simulink model "planner_contral"  (R2023b)
settings: Solver=FixedStepAuto  StartTime=0  StopTime=inf  FixedStep=0.001  RelTol=1e-3
undefined symbols (not defined in the file): aubr, c_factor, cf, cr, iniObsHeading1, iniObsHeading2, iniObsPos1, iniObsPos2, KD_PID_distance, KD_PID_speed, KI_PID_distance, KI_PID_speed, KP_PID_distance, KP_PID_speed, la, lb, LQR_K1, LQR_K2, LQR_K3, LQR_K4, m, rack_displacement, refInfo_obs1, refInfo_obs2, right_wheel_ground, rightWaypoints, tablebr, vubr, vx_break_point
libraries: Solver_SF x1
(part 4 of 8)

== matlab function planner_contral/decision_planning/EMplanner/obs/Cartesian2Frenet_dynamic/location transformer ==
  data: x_set input; s_set output; y_set input; frenet_path_x input; frenet_path_y input; proj_x_set input; proj_y_set input; proj_heading_set input; proj_match_point_index_set input; index2s input; l_set output
function [s_set,l_set] = fcn(x_set,y_set,frenet_path_x,frenet_path_y,...
    proj_x_set,proj_y_set,proj_heading_set,proj_match_point_index_set,index2s)
    %该函数将计算世界坐标系下的x_set，y_set上的点在frenet_path下的坐标s l
    %输入 x_set,y_set 待坐标转换的点
    %     frenet_path_x,frenet_path_y   frenet坐标轴
    %     proj_x,y,heading,kappa,proj_match_point_index 待坐标转换的点的投影点的信息
    %     index2s   frenet_path的index与s的转换表

    % 由于不知道有多少个点需要做坐标转换，所以需要做缓冲
    n = 128;%最多处理128个点
    %输出初始化
    s_set = ones(n,1)*nan;
    l_set = ones(n,1)*nan;
    for i = 1:length(x_set)
        if isnan(x_set(i))
            break;
        end
        %计算s，写个子函数
        s_set(i) = CalcSFromIndex2S(index2s,frenet_path_x,frenet_path_y,proj_x_set(i),proj_y_set(i),...
            proj_match_point_index_set(i));
        n_r = [-sin(proj_heading_set(i));cos(proj_heading_set(i))];
        r_h = [x_set(i);y_set(i)];
        r_r = [proj_x_set(i);proj_y_set(i)];
        l_set(i) = (r_h - r_r)'*n_r;
    end
end

function s = CalcSFromIndex2S(index2s,path_x,path_y,proj_x,proj_y,proj_match_point_index)
  %该函数将计算当指定index2s的映射关系后，计算点proj_x,proj_y的弧长
  vector_1 = [proj_x;proj_y] - [path_x(proj_match_point_index);path_y(proj_match_point_index)];
  %这里要考虑的更全面一些，因为要考虑到proj_match_point_index有可能在path的起点或终点
  if (proj_match_point_index < length(path_x))
      vector_2 = [path_x(proj_match_point_index + 1);path_y(proj_match_point_index + 1)] - ...
          [path_x(proj_match_point_index);path_y(proj_match_point_index)];
  else
      vector_2 = [path_x(proj_match_point_index);path_y(proj_match_point_index)] - ...
          [path_x(proj_match_point_index - 1);path_y(proj_match_point_index - 1)];
  end
  
  if vector_1'*vector_2 > 0
      s = index2s(proj_match_point_index) + sqrt(vector_1'*vector_1);
  else
      s = index2s(proj_match_point_index) - sqrt(vector_1'*vector_1);
  end
  
  
end

== matlab function planner_contral/decision_planning/EMplanner/obs/Cartesian2Frenet_dynamic/velocity transformer ==
  data: l_set input; s_dot_set output; vx_set input; vy_set input; proj_heading_set input; proj_kappa_set input; l_dot_set output; dl_set output
function [s_dot_set,l_dot_set,dl_set] = fcn(l_set,vx_set,vy_set,proj_heading_set,proj_kappa_set)
%该函数将计算frenet坐标系下的s_dot, l_dot, dl/ds
n = 128;
% 输出初始化
s_dot_set = ones(n,1)*nan;
l_dot_set = ones(n,1)*nan;
dl_set = ones(n,1)*nan;

for i = 1 : length(l_set)
    if isnan(l_set(i))
        break;
    end
    v_h = [vx_set(i);vy_set(i)];
    n_r = [-sin(proj_heading_set(i));cos(proj_heading_set(i))];
    t_r = [cos(proj_heading_set(i));sin(proj_heading_set(i))];
    l_dot_set(i) = v_h'*n_r;
    s_dot_set(i) = v_h'*t_r/(1 - proj_kappa_set(i)*l_set(i));
    %%%向量法做cartesian与frenet的转换要更简单，但是也有缺点，向量法必须依赖速度加速度
    %l' = l_dot/s_dot 但是如果s_dot = 0 此方法就失效了
    if abs(s_dot_set(i)) < 1e-6
        dl_set(i) = 0;
    else
        dl_set(i) = l_dot_set(i)/s_dot_set(i);
    end
end

== matlab function planner_contral/decision_planning/EMplanner/obs/Cartesian2Frenet_dynamic/acc transformer ==
  data: ax_set input; s_dot2_set output; ay_set input; proj_heading_set input; proj_kappa_set input; l_set input; s_dot_set input; dl_set input; l_dot2_set output; ddl_set output
function [s_dot2_set,l_dot2_set,ddl_set] = fcn(ax_set,ay_set,proj_heading_set,proj_kappa_set,l_set,s_dot_set,dl_set)
%由于不知道有多少个点需要做坐标转换，设一个最大值做缓冲
n = 128;
% 输出初始化
s_dot2_set = ones(n,1)*nan;
l_dot2_set = ones(n,1)*nan;
ddl_set = ones(n,1)*nan;

for i = 1:length(l_set)
    if isnan(l_set(i))
       break;
    end
    a_h = [ax_set(i);ay_set(i)];
    n_r = [-sin(proj_heading_set(i));cos(proj_heading_set(i))];
    t_r = [cos(proj_heading_set(i));sin(proj_heading_set(i))];
    %近似认为dkr/ds 为0 简化计算
    l_dot2_set(i) = a_h'*n_r - proj_kappa_set(i) * (1 - proj_kappa_set(i) * l_set(i)) * s_dot_set(i)^2;
    s_dot2_set(i) = (1/(1 - proj_kappa_set(i) * l_set(i)))* (a_h' * t_r + 2 * proj_kappa_set(i) * dl_set(i) * s_dot_set(i)^2);
    % 要考虑加速度为0的情况
    if (s_dot2_set(i) < 1e-6)
        ddl_set(i) = 0;
    else
        ddl_set(i) = (l_dot2_set(i) - dl_set(i)*s_dot2_set(i))/(s_dot_set(i)^2);
    end
end

== matlab function planner_contral/decision_planning/EMplanner/path planning task/generate convex space ==
  data: dp_path_s input; l_min output; dp_path_l input; static_obs_s_set input; static_obs_l_set input; dynamic_obs_s input; dynamic_obs_l input; dynamic_obs_heading input; l_max output; obs_length input; obs_width input
function [l_min,l_max] = fcn(dp_path_s,dp_path_l,static_obs_s_set,static_obs_l_set,dynamic_obs_s,dynamic_obs_l,dynamic_obs_heading,obs_length,obs_width)
    % 该函数将输出每个离散的dp_path_s所对应的l的边界lmin lmax (本质上是质点的凸空间)
    % 输入 动态规划曲线 dp_path_s,dp_path_l
    %      障碍物中心的s l 坐标 static_obs_s,static_obs_l
    %      障碍物的长宽 static_obs_length,static_obs_width 
    % 输出 l_min lmax l 的上下界

    % 输出初始化
    l_min = ones(60,1) * -8;
    l_max = ones(60,1) * 8;
    % 对每个静态障碍物做遍历
    for i = 1:length(static_obs_s_set)
        if isnan(static_obs_s_set(i))
            break;
        end
        % 计算障碍物的头部和尾部的s
        obs_s_min = static_obs_s_set(i) - obs_length/2;
        obs_s_max = static_obs_s_set(i) + obs_length/2;
        % 找到dp_path_s 中，与s_head s_end最近的s的编号
        start_index = FindNearIndex(dp_path_s,obs_s_min);
        end_index = FindNearIndex(dp_path_s,obs_s_max);
        path_l = (dp_path_l(start_index) + dp_path_l(end_index))/2;
        if start_index == 1 && end_index == 1
            continue;
        end
        if path_l > static_obs_l_set(i)
            % 意味着决策为向左绕过障碍物
            for j = start_index:end_index
                % l_min(j) 为所有决策为向左绕过障碍物的l边界的最大值
                l_min(j) = max(l_min(j) , static_obs_l_set(i) + obs_width/2+0.6);
            end
        else
            % 意味着决策为向右绕过障碍物
            for j = start_index:end_index
                % l_max(j) 为所有决策为向右绕过障碍物的l边界的最小值
                l_max(j) = min(l_max(j) ,static_obs_l_set(i) - obs_width/2-0.6);
            end
        end       
    end
%计算动态障碍物的上界与下界
for i=1:length(dynamic_obs_s)
    if isnan(dynamic_obs_s(i))
        break;
    end
    %计算障碍物的头和尾，通过障碍物的坐标点及其航向角计算
%         obs_s_min = dynamic_obs_s(i) - obs_length/2;
%         obs_s_max = dynamic_obs_s(i) + obs_length/2;
        [l_max_,l_min_,s_max_,s_min_]=getboxpoint(dynamic_obs_s(i),dynamic_obs_l(i),dynamic_obs_heading(i),obs_length,obs_width);
        obs_s_min =s_min_;
        obs_s_max=s_max_;
        obs_l_min=l_min_;
        obs_l_max=l_max_;
        start_index = FindNearIndex(dp_path_s,obs_s_min);
        end_index = FindNearIndex(dp_path_s,obs_s_max);
        path_l = (dp_path_l(start_index) + dp_path_l(end_index))/2;
        if start_index == 1 && end_index == 1
            continue;
        end
         if path_l > dynamic_obs_l(i)
            % 意味着决策为向左绕过障碍物
            for j = start_index:end_index
                % l_min(j) 为所有决策为向左绕过障碍物的l边界的最大值dynamic_obs_l(i) + obs_width/2)+0.2
                l_min(j) = max(l_min(j) , obs_l_max+0.6);   %如果此l_min有数值，以最大值替代，但有个问题就是障碍物有航向。
            end
        else
            % 意味着决策为向右绕过障碍物
            for j = start_index:end_index
                % l_max(j) 为所有决策为向右绕过障碍物的l边界的最小值dynamic_obs_l(i) - obs_width/2)-0.2
                l_max(j) = min(l_max(j) , obs_l_min-0.6);
            end
        end       
 end


end

function y = FindNearIndex(dp_path_s,obs_s)
    % 该函数将找到dp_path_s的所有点中，距离obs_s最近的点的编号
    % 这里要注意obs_s 是在完整的reference line上投影所得到的坐标，所以obs_s可能是负值，也可能会超过dp_path_s最远的长度
    if dp_path_s(1) >= obs_s
        %障碍物在后面
        y = 1;
        return;
    elseif dp_path_s(end) <= obs_s
        y = 60;
        return;
    else
        index = 1;
        while dp_path_s(index) < obs_s
            index = index + 1;
        end
        % 循环退出的条件是dp_path_s(index) >= obs_s 判断一下index 和 index-1哪个离的近
        if dp_path_s(index) - obs_s > obs_s - dp_path_s(index - 1)
            y = index - 1;
        else
            y = index;
        end
    end
end
%该函数计算车辆四个角点的最大值
function [l_max,l_min,s_max,s_min]=getboxpoint(obs_s,obs_l,obs_heading,obs_length,obs_width)
%获取车辆后轴中心点
    l_set=zeros(4,1);
    s_set=zeros(4,1);
    rear_s = obs_s;
    rear_l = obs_l;
%计算前轴中心点
    front_s=rear_s+obs_length*cos(obs_heading);
    front_l=rear_l+obs_length*sin(obs_heading);
 %计算四个角点的的l及s
    l_ringht_upper=front_l+obs_width/2*cos(obs_heading);
    s_ringht_upper=front_s-obs_width/2*sin(obs_heading);

    l_right_low=front_l-obs_width/2*cos(obs_heading);
    s_right_low=front_s+obs_width/2*sin(obs_heading);

    l_left_upper=rear_l+obs_width/2*cos(obs_heading);
    s_left_upper=rear_s-obs_width/2*sin(obs_heading);

    l_left_low=rear_l-obs_width/2*cos(obs_heading);
    s_left_low= rear_s+obs_width/2*sin(obs_heading);
 

    l_set(1)= l_ringht_upper;
    l_set(2)=l_right_low;
    l_set(3)=l_left_upper;
    l_set(4)=l_left_low;
    s_set(1)= s_ringht_upper;
    s_set(2)=s_right_low;
    s_set(3)=s_left_upper;
    s_set(4)=s_left_low;
    l_max=max(l_set);
    l_min=min(l_set);
    s_max=max(s_set);
    s_min=min(s_set);

end

== matlab function planner_contral/decision_planning/EMplanner/path planning task/path planning with quadratic programming (qp) ==
  data: qp_path_s output; l_min input; qp_path_l output; l_max input; w_cost_l input; w_cost_dl input; w_cost_ddl input; w_cost_dddl input; w_cost_centre input; w_cost_end_l input; w_cost_end_dl input; w_cost_end_ddl input; w_ref_dp input; host_d1 input; host_d2 input; host_w input; plan_start_s input; plan_start_l input; plan_start_dl input; plan_start_ddl input; qp_path_dl output; qp_path_ddl output; delta_dl_max input; delta_ddl_max input; dp_path_l_final input
function [qp_path_s,qp_path_l,qp_path_dl,qp_path_ddl] = ...
fcn(l_min,l_max,w_cost_l,w_cost_dl,w_cost_ddl,w_cost_dddl,w_cost_centre,w_cost_end_l,w_cost_end_dl,w_cost_end_ddl,w_ref_dp,...
    host_d1,host_d2,host_w,...
    plan_start_s,plan_start_l,plan_start_dl,plan_start_ddl,...
    delta_dl_max,delta_ddl_max,dp_path_l_final)
% 路径二次规划
% 0.5*x'Hx + f'*x = min
% subject to A*x <= b
%            Aeq*x = beq
%            lb <= x <= ub;
% 输入：l_min l_max 点的凸空间
%       w_cost_l 参考线代价
%       w_cost_dl ddl dddl 光滑性代价
%       w_cost_centre 凸空间中央代价
%       w_cost_end_l dl dd1 终点的状态代价 (希望path的终点状态为(0,0,0))
%       host_d1,d2 host质心到前后轴的距离
%       host_w host的宽度
%       plan_start_l,dl,ddl 规划起点
% 输出 qp_path_l dl ddl 二次规划输出的曲线
coder.extrinsic("quadprog");
% 待优化的变量的数量QP 只在 20 个离散点上优化。
% 每个点优化3个变量
n = 20;

% 输出初始化
qp_path_l = zeros(n,1);
qp_path_dl = zeros(n,1);
qp_path_ddl = zeros(n,1);
qp_path_s = zeros(n,1);

% H_L H_DL H_DDL H_DDDL Aeq beq A b 初始化
H_L = zeros(3*n, 3*n);
H_DL = zeros(3*n, 3*n);
H_DDL = zeros(3*n, 3*n);
H_DDDL = zeros(n-1, 3*n);
H_CENTRE = zeros(3*n, 3*n);
H_L_END = zeros(3*n, 3*n);
H_DL_END = zeros(3*n, 3*n);
H_DDL_END = zeros(3*n, 3*n);
H_REF_DP= zeros(3*n, 3*n);
Aeq = zeros(2*n-2, 3*n);
beq = zeros(2*n-2, 1);
A = zeros(8*n, 3*n);
b = zeros(8*n, 1);
% 更新：加入 dl(i+1) - dl(i) ddl(i+1) - ddl(i) 的约束
A_dl_minus = zeros(n - 1,3*n);
b_dl_minus = zeros(n - 1,1);
A_ddl_minus = zeros(n - 1,3*n);
b_ddl_minus = zeros(n - 1,1);
for i = 1:n-1
    row = i;
    col = 3*i - 2;
    A_dl_minus(row,col:col+5) = [0 -1 0 0 1 0];
    b_dl_minus(row) = delta_dl_max;
    A_ddl_minus(row,col:col+5) = [0 0 -1 0 0 1];
    b_ddl_minus(row) = delta_ddl_max;
end
% -max < a*x < max => ax < max && -ax < -(-max)
A_minus = [A_dl_minus;
          -A_dl_minus;
           A_ddl_minus;
          -A_ddl_minus];
b_minus = [b_dl_minus;
           b_dl_minus;
          b_ddl_minus;
          b_ddl_minus]; 

%  期望的终点状态
end_l_desire = 0;
end_dl_desire = 0;
end_ddl_desire = 0;

% Aeq_sub
ds = 3;%纵向间隔
for i = 1:n
    qp_path_s(i) = plan_start_s + (i-1)*ds;
end

Aeq_sub = [1 ds ds^2/3 -1 0 ds^2/6;
           0 1  ds/2   0 -1 ds/2];
% A_sub;
d1 = host_d1;
d2 = host_d2;
w = host_w;
A_sub = [1  d1 0;
         1  d1 0;
         1 -d2 0;
         1 -d2 0;
        -1 -d1 0;
        -1 -d1 0;
        -1  d2 0;
        -1  d2 0];
% 生成Aeq
for i = 1:n-1
    % 计算分块矩阵左上角的行和列
    row = 2*i - 1;
    col = 3*i - 2;
    Aeq(row:row + 1,col:col + 5) = Aeq_sub;
end
% 生成A
for i = 2:n
    row = 8*i - 7;
    col = 3*i - 2;
    A(row:row + 7,col:col + 2) = A_sub;
end

% 视频里用的找(s(i) - d2,s(i) + d1)的方法过于保守，在这里舍弃掉
% 只要找到四个角点所对应的l_min l_max 即可
% 。。。。。。。。。。。。。。
%    [    .   ]<- 
%    [        ]
% 。。。。。。。。。。。。。
front_index = ceil(d1/ds);
back_index = ceil(d2/ds); % ceil向上取整 ceil(3) = 3 ceil(3.1) = 4
% 生成b
for i = 2:n
    % 左前 右前的index = min(i + front_index,60)
    % 左后 右后的index = max(i - back_index,1)
    % l_min l_max 都是60个点
    index1 = min(3*i - 2 + front_index,n);
    index2 = max(3*i - 2 - back_index,1);
    b(8*i - 7:8*i,1) = [l_max(index1) - w/2;
                        l_max(index1) + w/2;
                        l_max(index2) - w/2;
                        l_max(index2) + w/2;
                       -l_min(index1) + w/2;
                       -l_min(index1) - w/2;
                       -l_min(index2) + w/2;
                       -l_min(index2) - w/2;];
end
%生成 lb ub 主要是对规划起点做约束
lb = ones(3*n,1)*-inf;
ub = ones(3*n,1)*inf;
lb(1) = plan_start_l;
lb(2) = plan_start_dl;
lb(3) = plan_start_ddl;
ub(1) = lb(1);
ub(2) = lb(2);
ub(3) = lb(3);
%应该多约束L
for i = 2:n
    lb(3*i - 1) = - 1; %约束 l'
    ub(3*i - 1) = 1;
    lb(3*i) = -0.1; %约束 l''
    ub(3*i) = 0.1;
end
% 生成H_L,H_DL,H_DDL,H_CENTRE
for i = 1:n
    H_L(3*i - 2,3*i - 2) = 1;
    H_DL(3*i - 1,3*i - 1) = 1;
    H_DDL(3*i, 3*i) = 1;
    H_REF_DP(3*i-2, 3*i-2)=1;
end
H_CENTRE = H_L;
% 生成H_DDDL;
H_dddl_sub = [0 0 1 0 0 -1];
for i = 1:n-1
    row = i;
    col = 3*i - 2;
    H_DDDL(row,col:col + 5) = H_dddl_sub;
end
% 生成H_L_END H_DL_END H_DDL_END
H_L_END(3*n - 2,3*n - 2) = 1;
H_DL_END(3*n - 1,3*n - 1) = 1;
H_DDL_END(3*n,3*n) = 1;
% 生成二次规划的H 因为ds ！= 1 所以 dddl = delta_ddl/ds;
H = w_cost_l * (H_L'*H_L) + w_cost_dl * (H_DL'*H_DL) + w_cost_ddl * (H_DDL'*H_DDL)...
   +w_cost_dddl * (H_DDDL'*H_DDDL)/ds + w_cost_centre * (H_CENTRE'*H_CENTRE) + w_cost_end_l * (H_L_END'*H_L_END)...
   +w_cost_end_dl * (H_DL_END'* H_DL_END) + w_cost_ddl * (H_DDL_END'*H_DDL_END)+w_ref_dp*(H_REF_DP'*H_REF_DP);
H = 2 * H;
% 生成f
f = zeros(3*n,1);
 centre_line = 0.5 * (l_min + l_max); % 此时centre line 还是60个点
% centre_line = dp_path_l_final;
for i = 1:n
    f(3*i - 2) = -2 * centre_line(3*i - 2);
     f(3*i - 2) = -2 *w_ref_dp*dp_path_l_final(3*i);
end
% 避免centreline权重过大影响轨迹平顺性
for i = 1:n
    if abs(f(i)) > 0.5
        f(i) = w_cost_centre * f(i);
    end
end
% 终点要接近end_l dl ddl desire
f(3*n - 2) = f(3*n - 2) -2 * end_l_desire * w_cost_end_l;
f(3*n - 1) = f(3*n - 1) -2 * end_dl_desire * w_cost_end_dl;
f(3*n) = f(3*n) -2 * end_ddl_desire * w_cost_end_ddl;

X = quadprog(H,f,[A;A_minus],[b;b_minus],Aeq,beq,lb,ub);

for i = 1:n
    qp_path_l(i) = X(3*i - 2);
    qp_path_dl(i) = X(3*i - 1);
    qp_path_ddl(i) = X(3*i);
end

end

== matlab function planner_contral/decision_planning/EMplanner/obs/000 ==
  data: dynamic_obs_x_set_gcs input; dynamic_obs_y_set_gcs input; dynamic_obs_heading_set_gcs input; dynamic_obs_velocity_set_gcs input; dynamic_obs1_x_pre output; dynamic_obs1_y_pre output; dynamic_obs1_vx_set output; dynamic_obs1_vy_set output; pre_obs1 input
function [dynamic_obs1_x_pre, dynamic_obs1_y_pre, dynamic_obs1_vx_set, dynamic_obs1_vy_set] = ...
    fcn(dynamic_obs_x_set_gcs, dynamic_obs_y_set_gcs, dynamic_obs_heading_set_gcs, dynamic_obs_velocity_set_gcs, pre_obs1)

% 生成当前有效动态障碍物的预测轨迹。
% 当前模型下游只支持一条动态障碍物轨迹，因此这里选取筛选后的第一个动态障碍物。
% 如果该障碍物与 pre_obs1 起点匹配，则使用 pre_obs1；
% 否则使用当前速度做匀速预测，避免 obs2 错误拼接 obs1 预测轨迹。

n = 32;
dt = 0.1;
match_threshold = 5.0;

dynamic_obs1_x_pre = nan(n, 1);
dynamic_obs1_y_pre = nan(n, 1);
dynamic_obs1_vx_set = nan(n, 1);
dynamic_obs1_vy_set = nan(n, 1);

idx = 0;
for i = 1:length(dynamic_obs_x_set_gcs)
    if ~isnan(dynamic_obs_x_set_gcs(i)) && ~isnan(dynamic_obs_velocity_set_gcs(i))
        idx = i;
        break;
    end
end

if idx == 0
    return;
end

x0 = dynamic_obs_x_set_gcs(idx);
y0 = dynamic_obs_y_set_gcs(idx);
heading = dynamic_obs_heading_set_gcs(idx);
speed = dynamic_obs_velocity_set_gcs(idx);

vx = speed * cos(heading);
vy = speed * sin(heading);

dynamic_obs1_x_pre(1) = x0;
dynamic_obs1_y_pre(1) = y0;
dynamic_obs1_vx_set(1) = vx;
dynamic_obs1_vy_set(1) = vy;

use_pre_obs1 = false;
if ~isempty(pre_obs1) && size(pre_obs1, 2) >= 2 && all(isfinite(pre_obs1(1, 1:2)))
    dist_to_pre1 = hypot(x0 - pre_obs1(1, 1), y0 - pre_obs1(1, 2));
    use_pre_obs1 = dist_to_pre1 < match_threshold;
end

if use_pre_obs1
    m = min(size(pre_obs1, 1), n - 1);
    for j = 1:m
        dynamic_obs1_x_pre(j + 1) = pre_obs1(j, 1);
        dynamic_obs1_y_pre(j + 1) = pre_obs1(j, 2);
        dynamic_obs1_vx_set(j + 1) = vx;
        dynamic_obs1_vy_set(j + 1) = vy;
    end
else
    for j = 2:n
        t = (j - 1) * dt;
        dynamic_obs1_x_pre(j) = x0 + vx * t;
        dynamic_obs1_y_pre(j) = y0 + vy * t;
        dynamic_obs1_vx_set(j) = vx;
        dynamic_obs1_vy_set(j) = vy;
    end
end
end

== matlab function planner_contral/decision_planning/EMplanner/obs/111 ==
  data: x_set input; match_point_index_set output; y_set input; frenet_path_x input; frenet_path_y input; frenet_path_heading input; frenet_path_kappa input; proj_x_set output; proj_y_set output; proj_heading_set output; proj_kappa_set output
function [match_point_index_set,proj_x_set, proj_y_set,proj_heading_set,proj_kappa_set] = ...
    fcn(x_set,y_set,frenet_path_x,frenet_path_y,frenet_path_heading,frenet_path_kappa)
%该函数将批量计算x_set，y_set中的xy，在frenet_path下的投影的信息
%输入 x_set,y_set，待投影的点的集合
%x_set,y_set,frenet_path_x,frenet_path_y,frenet_path_heading,frenet_path_kappa
%曲线在直角坐标系下的x，y，heading，kappa
%输出：match_point_index_set 匹配点在frenet_path下的编号的集合(即从全局路径第一个点开始数，第几个点是匹配点)
%     proj_x y heading kappa 投影的x,y,heading,kappa的集合

% 由于事先不知道x_set中到底有多少个点需要投影，因此事先声明一个最大的数量的点作为缓冲
n = 128;
% 并且由于不知道投影点的个数，所以也不知道输出的个数，因此输出也要做缓冲，用nan表示不存在的点
% 输出最多输出128个
% 输出初始化
match_point_index_set = ones(n,1) * nan;
proj_x_set = ones(n,1) * nan;
proj_y_set = ones(n,1) * nan;
proj_heading_set = ones(n,1) * nan;
proj_kappa_set = ones(n,1) * nan;

% 找匹配点，需要利用上一个周期的结果作为下一个周期遍历的起点，因此需要声明两个全局变量

persistent is_first_run;
persistent pre_match_point_index_set;%bug :pre_match_point_index(i) 未必代表的是第i个障碍物的match_point_index
persistent pre_frenet_path_x;
persistent pre_frenet_path_y;
persistent pre_frenet_path_heading;
persistent pre_frenet_path_kappa;
persistent pre_x_set;
persistent pre_y_set;
%算法主函数入口

if isempty(is_first_run)
    %该if分支表示函数首次运行
    is_first_run = 0;
    pre_frenet_path_x = frenet_path_x;
    pre_frenet_path_y = frenet_path_y;
    pre_frenet_path_heading = frenet_path_heading;
    pre_frenet_path_kappa = frenet_path_kappa;
    %要记录首次运行计算的匹配点的结果供下个周期运行，先初始化
    pre_match_point_index_set = ones(n,1) * nan;
    %对x_set,y_set的点做遍历，找到他们的匹配点
    for i = 1 : length(x_set)
        if isnan(x_set(i))
            break;
        end
        %首次运行时，没有任何提示，只能从frenet path的第一个点开始找
        start_search_index = 1;
        % 声明increase_count，用于表示在遍历时distance连续增加的个数
        increase_count = 0;
        % 开始遍历
        min_distance = inf;
        for j = start_search_index : length(frenet_path_x)
            distance = (x_set(i) - frenet_path_x(j))^2 + (y_set(i) - frenet_path_y(j))^2;
            if distance < min_distance
                min_distance = distance;
                match_point_index_set(i) = j;
                increase_count = 0;
            else
                increase_count = increase_count + 1;
            end
            %如果distance连续增加50次就不要再遍历了，节省时间
            if increase_count > 50
                break;
            end
        end
        
        %如何通过匹配点计算投影点，请参见《自动驾驶控制算法第七讲》
        %或《自动驾驶决策规划算法》第一章第三节
        
        %取出匹配点的编号
        match_point_index = match_point_index_set(i);
        %取出匹配点的信息
        match_point_x = frenet_path_x(match_point_index);
        match_point_y = frenet_path_y(match_point_index);
        match_point_heading = frenet_path_heading(match_point_index);
        match_point_kappa = frenet_path_kappa(match_point_index);
        %计算匹配点的方向向量与法向量
        vector_match_point = [match_point_x;match_point_y];
        vector_match_point_direction = [cos(match_point_heading);sin(match_point_heading)];
        %声明待投影点的位矢
        vector_r = [x_set(i);y_set(i)];
        
       %通过匹配点计算投影点
       vector_d = vector_r - vector_match_point;
       ds = vector_d' * vector_match_point_direction;
       vector_proj_point = vector_match_point + ds * vector_match_point_direction;
       proj_heading = match_point_heading + match_point_kappa * ds;
       proj_kappa = match_point_kappa;
       %计算结果输出
       proj_x_set(i) = vector_proj_point(1);
       proj_y_set(i) = vector_proj_point(2);
       proj_heading_set(i) = proj_heading;
       proj_kappa_set(i) = proj_kappa;
    end
    %匹配点的计算结果保存，供下一个周期使用
    pre_match_point_index_set = match_point_index_set;
    pre_x_set = x_set;
    pre_y_set = y_set;
else
    %此if分支表示不是首次运行
    %对每个x_set上的点做处理
    for i = 1 : length(x_set)
        %不是首次运行，对于点x_set(i),y_set(i)来说,start_search_index =
        %pre_match_point_index_set(i)
        start_search_index = pre_match_point_index_set(i);%上个周期匹配点的编号作为本周期搜索的起点
        % 判断帧与帧之间的障碍物是否为同一个
        square_dis = (x_set(i) - pre_x_set(i))^2 + (y_set(i) - pre_y_set(i))^2;
        if square_dis > 36
            % 帧与帧之间的物体的位置距离过大，认为是两个障碍物
            start_search_index = nan;
        end
        % 声明increase_count，用于表示在遍历时distance连续增加的个数
        %%%%%%%%%
        %对于障碍物检测而言，当感知第一次检测到障碍物时，算法并不是首次运行，此时 
        %pre_match_point_index_set的值是nan，如果还用上一时刻的结果作为本周期搜索的起点
        %必然会出问题，所以要修改
        % 声明increase_count_limit
        increase_count_limit = 5;
        if isnan(start_search_index)
            %没有上个周期的结果，那就不能只检查5次了
            increase_count_limit = 50;
            %搜索起点也要设为1
            start_search_index = 1;
        end
        increase_count = 0;
        % 开始遍历
        %这里多一个步骤，判断遍历的方向
        %计算上个周期匹配点的位矢
        vector_pre_match_point = [pre_frenet_path_x(start_search_index);pre_frenet_path_y(start_search_index)];
        vector_pre_match_point_direction = ...
            [cos(pre_frenet_path_heading(start_search_index));sin(pre_frenet_path_heading(start_search_index))];
        %判断遍历的方向
        flag = ([x_set(i);y_set(i)] - vector_pre_match_point)' * vector_pre_match_point_direction;
        min_distance = inf;
        if flag > 0.001
            for j = start_search_index : length(frenet_path_x)
                distance = (x_set(i) - frenet_path_x(j))^2 + (y_set(i) - frenet_path_y(j))^2;
                if distance < min_distance
                    min_distance = distance;
                    match_point_index_set(i) = j;
                    increase_count = 0;
                else
                    increase_count = increase_count + 1;
                end
                %如果distance连续增加increase_count_limit次就不要再遍历了，节省时间
                if increase_count > increase_count_limit
                    break;
                end
            end
        elseif flag < - 0.001
            for j = start_search_index : -1 : 1
                distance = (x_set(i) - frenet_path_x(j))^2 + (y_set(i) - frenet_path_y(j))^2;
                if distance < min_distance
                    min_distance = distance;
                    match_point_index_set(i) = j;
                    increase_count = 0;
                else
                    increase_count = increase_count + 1;
                end
                %如果distance连续增加increase_count_limit次就不要再遍历了，节省时间
                if increase_count > increase_count_limit
                    break;
                end
            end
        else
            match_point_index_set(i) = start_search_index;
        end
        
        %如何通过匹配点计算投影点，请参见《自动驾驶控制算法第七讲》
        %或《自动驾驶决策规划算法》第一章第三节
        
        %取出匹配点的编号
        match_point_index = match_point_index_set(i);
        %取出匹配点的信息
        match_point_x = frenet_path_x(match_point_index);
        match_point_y = frenet_path_y(match_point_index);
        match_point_heading = frenet_path_heading(match_point_index);
        match_point_kappa = frenet_path_kappa(match_point_index);
        %计算匹配点的方向向量与法向量
        vector_match_point = [match_point_x;match_point_y];
        vector_match_point_direction = [cos(match_point_heading);sin(match_point_heading)];
        %声明待投影点的位矢
        vector_r = [x_set(i);y_set(i)];
        
       %通过匹配点计算投影点
       vector_d = vector_r - vector_match_point;
       ds = vector_d' * vector_match_point_direction;
       vector_proj_point = vector_match_point + ds * vector_match_point_direction;
       proj_heading = match_point_heading + match_point_kappa * ds;
       proj_kappa = match_point_kappa;
       %计算结果输出
       proj_x_set(i) = vector_proj_point(1);
       proj_y_set(i) = vector_proj_point(2);
       proj_heading_set(i) = proj_heading;
       proj_kappa_set(i) = proj_kappa;
  
    end
    %匹配点的计算结果保存，供下一个周期使用
    pre_match_point_index_set = match_point_index_set;
    pre_frenet_path_x = frenet_path_x;
    pre_frenet_path_y = frenet_path_y;
    pre_frenet_path_heading = frenet_path_heading;
    pre_frenet_path_kappa = frenet_path_kappa;
    pre_x_set = x_set;
    pre_y_set = y_set;
end

== matlab function planner_contral/decision_planning/EMplanner/generate convex space ==
  data: dp_speed_s input; s_lb output; dp_speed_t input; path_index2s input; static_obs_s_lb input; static_obs_s_ub input; static_obs_t_lb input; static_obs_t_ub input; dynamic_obs_s_lb input; dynamic_obs_s_ub input; dynamic_obs_t_lb input; dynamic_obs_t_ub input; s_ub output; s_dot_lb output; s_dot_ub output; trajectory_kappa_init input; max_lateral_accel input; static_s_ub output; static_s_lb output
%% 基于 DP 粗速度解的连续双边 ST 可行域重构
% 作用：
% 1. 根据 DP 粗解生成 QP 的 s 方向双边约束
% 2. 根据静态/动态障碍物 ST 边界裁剪可行域
% 3. 修复边界退化、可行域过窄、局部动力学不可达等问题
% 4. 输出 QP 速度规划需要的 s_lb/s_ub/s_dot_lb/s_dot_ub

function [s_lb,s_ub,s_dot_lb,s_dot_ub, static_s_ub,static_s_lb] = fcn( ...
    dp_speed_s,dp_speed_t,path_index2s, ...
    static_obs_s_lb,static_obs_s_ub,static_obs_t_lb,static_obs_t_ub, ...
    dynamic_obs_s_lb,dynamic_obs_s_ub,dynamic_obs_t_lb,dynamic_obs_t_ub, ...
    trajectory_kappa_init,max_lateral_accel)

n = 16;

safe_margin = 1.0;        % 障碍物纵向安全距离
back_margin = 10.0;       % DP 曲线后方保留距离
front_margin = 14.0;      % DP 曲线前方保留距离
min_width = 6.0;          % 期望可行域宽度；不能为了满足它而侵入障碍物硬边界
s_floor = 0.0;            % 局部 s 下界
default_speed_ub = 30.0;  % 默认速度上界

acc_min = -6.0;           % 最小加速度
acc_max = 4.0;            % 最大加速度

% QP 速度规划采样点：0.5s 到 8s
t_qp = (0.5:0.5:8.0)';

% ST 图时间采样点：0s 到 8s，间隔 0.1s
t_st = (0:0.1:8.0)';

% ============================================================
% 输出初始化
% ============================================================
s_lb = zeros(n,1);
s_ub = zeros(n,1);

static_s_lb = ones(n,1) * -inf;
static_s_ub = ones(n,1) * inf;

s_dot_lb = zeros(n,1);
s_dot_ub = ones(n,1) * default_speed_ub;

% hard_lb/hard_ub 是障碍物 ST 安全边界，后续任何修复都不能越过它。
hard_lb = ones(n,1) * -inf;
hard_ub = ones(n,1) * inf;

% ============================================================
% 整理 DP 粗速度解
% ============================================================
valid_dp = isfinite(dp_speed_s) & isfinite(dp_speed_t);
dp_s_valid = dp_speed_s(valid_dp);
dp_t_valid = dp_speed_t(valid_dp);

if isempty(dp_s_valid)
    % 如果 DP 没有有效解，则给一个保守但不崩溃的默认可行域
    for i = 1:n
        s_lb(i) = s_floor;
        s_ub(i) = front_margin + 5.0 * i;
    end

    s_dot_ub = ones(n,1) * default_speed_ub;
    return;
end

% 保证 DP 时间单调
[dp_t_valid, order] = sort(dp_t_valid);
dp_s_valid = dp_s_valid(order);

% 去掉重复时间点，避免 interp1 出错
[dp_t_valid, uniqueIdx] = unique(dp_t_valid, 'stable');
dp_s_valid = dp_s_valid(uniqueIdx);

% 将 DP 粗解插值到 QP 采样点
s_dp_qp = interpHold(dp_t_valid, dp_s_valid, t_qp);

% ============================================================
% 以 DP 曲线为中心，初始化双边可行域
% ============================================================
for i = 1:n
    s_lb(i) = max(s_floor, s_dp_qp(i) - back_margin);
    s_ub(i) = s_dp_qp(i) + front_margin;
end

% ============================================================
% 收集静态障碍物硬边界
% ============================================================
for i = 1:n
    [obs_lb, obs_ub, has_obs] = getObstacleBoundAtTime( ...
        t_qp(i), t_st, static_obs_s_lb, static_obs_s_ub);

    if has_obs
        static_s_lb(i) = obs_lb;
        static_s_ub(i) = obs_ub;

        [hard_lb(i), hard_ub(i)] = updateHardBoundByObstacle( ...
            hard_lb(i), hard_ub(i), s_dp_qp(i), obs_lb, obs_ub, safe_margin);
    end
end

% ============================================================
% 收集动态障碍物硬边界
% ============================================================
for i = 1:n
    [obs_lb, obs_ub, has_obs] = getObstacleBoundAtTime( ...
        t_qp(i), t_st, dynamic_obs_s_lb, dynamic_obs_s_ub);

    if has_obs
        [hard_lb(i), hard_ub(i)] = updateHardBoundByObstacle( ...
            hard_lb(i), hard_ub(i), s_dp_qp(i), obs_lb, obs_ub, safe_margin);
    end
end

% 首次应用硬边界，得到安全侧的基础可行域。
for i = 1:n
    [s_lb(i), s_ub(i)] = repairCorridorInsideHardBounds( ...
        s_lb(i), s_ub(i), s_dp_qp(i), hard_lb(i), hard_ub(i), ...
        s_floor, front_margin, min_width);
end

% ============================================================
% 动力学可达性修复
% 说明：
% 当前函数接口没有 plan_start_s_dot 和 plan_start_s_dot2，
% 所以这里用 DP 曲线估计一个可达参考。修复过程中始终受 hard_lb/hard_ub 限制。
% ============================================================
[s_lb, s_ub] = repairReachableCorridor( ...
    s_lb, s_ub, s_dp_qp, hard_lb, hard_ub, ...
    acc_min, acc_max, min_width, s_floor, front_margin);

% ============================================================
% 最终硬边界再投影
% 这是本次修复的核心：所有连续性/宽度/可达性修复之后，
% 必须重新裁剪到静态/动态障碍物 ST 安全边界内。
% 这里不再强制 s_ub 非递减，因为动态障碍物进入窗口时，上界本来就应该下降。
% ============================================================
for i = 1:n
    [s_lb(i), s_ub(i)] = repairCorridorInsideHardBounds( ...
        s_lb(i), s_ub(i), s_dp_qp(i), hard_lb(i), hard_ub(i), ...
        s_floor, front_margin, min_width);

    if isfinite(hard_lb(i))
        s_lb(i) = max(s_lb(i), hard_lb(i));
    end

    if isfinite(hard_ub(i))
        s_ub(i) = min(s_ub(i), hard_ub(i));
    end

    % 如果硬边界导致区间很窄，优先保持安全，只给 QP 一个数值上可接受的窄区间。
    if s_ub(i) <= s_lb(i)
        if isfinite(hard_ub(i))
            s_ub(i) = hard_ub(i);
            s_lb(i) = max(s_floor, s_ub(i) - 0.1);
        else
            s_ub(i) = s_lb(i) + 0.1;
        end
    end
end

% ============================================================
% 速度上下界
% ============================================================
s_dot_lb = zeros(n,1);
s_dot_ub = ones(n,1) * default_speed_ub;

end

%% 根据 DP 粗解选择从障碍物前方还是后方通过，并更新硬边界
% s_dp < obs_lb：DP 在障碍物后方，约束上界
% s_dp > obs_ub：DP 在障碍物前方，约束下界
% s_dp 在障碍物内部：选择修正量较小的一侧
function [new_hard_lb, new_hard_ub] = updateHardBoundByObstacle( ...
    cur_hard_lb, cur_hard_ub, s_dp, obs_lb, obs_ub, safe_margin)

new_hard_lb = cur_hard_lb;
new_hard_ub = cur_hard_ub;

if ~isfinite(obs_lb) || ~isfinite(obs_ub)
    return;
end

if obs_ub < obs_lb
    temp = obs_lb;
    obs_lb = obs_ub;
    obs_ub = temp;
end

if s_dp < obs_lb
    new_hard_ub = min(new_hard_ub, obs_lb - safe_margin);
elseif s_dp > obs_ub
    new_hard_lb = max(new_hard_lb, obs_ub + safe_margin);
else
    dist_to_lb = abs(s_dp - obs_lb);
    dist_to_ub = abs(s_dp - obs_ub);

    if dist_to_lb <= dist_to_ub
        new_hard_ub = min(new_hard_ub, obs_lb - safe_margin);
    else
        new_hard_lb = max(new_hard_lb, obs_ub + safe_margin);
    end
end

end

%% 将可行域修复到硬边界内部
function [lb, ub] = repairCorridorInsideHardBounds( ...
    lb, ub, s_dp, hard_lb, hard_ub, s_floor, front_margin, min_width)

if ~isfinite(lb)
    lb = max(s_floor, s_dp - 0.5 * min_width);
end

if ~isfinite(ub)
    ub = s_dp + front_margin;
end

lb = max(lb, s_floor);

if isfinite(hard_lb)
    lb = max(lb, hard_lb);
end

if isfinite(hard_ub)
    ub = min(ub, hard_ub);
end

% 只在不破坏硬边界的前提下尝试扩宽。
if ub <= lb + min_width
    if isfinite(hard_lb) && isfinite(hard_ub)
        hard_width = hard_ub - hard_lb;
        if hard_width >= min_width
            center = min(max(s_dp, hard_lb + 0.5 * min_width), hard_ub - 0.5 * min_width);
            lb = center - 0.5 * min_width;
            ub = center + 0.5 * min_width;
        else
            lb = hard_lb;
            ub = hard_ub;
        end
    elseif isfinite(hard_ub)
        ub = hard_ub;
        lb = max(s_floor, ub - min_width);
    elseif isfinite(hard_lb)
        lb = hard_lb;
        ub = lb + min_width;
    else
        center = max(s_floor + 0.5 * min_width, s_dp);
        lb = max(s_floor, center - 0.5 * min_width);
        ub = lb + min_width;
    end
end

if isfinite(hard_lb)
    lb = max(lb, hard_lb);
end

if isfinite(hard_ub)
    ub = min(ub, hard_ub);
end

end

%% 从 ST 图中读取指定时间 t 对应的障碍物 s 边界
function [obs_lb, obs_ub, has_obs] = getObstacleBoundAtTime(t, t_grid, obs_lb_set, obs_ub_set)

obs_lb = inf;
obs_ub = -inf;
has_obs = false;

obs_min_width = 5.0;      % 障碍物 ST 纵向最小占用宽度
single_t_window = 0.25;   % 单点 ST 障碍物的时间保持窗口

valid = isfinite(obs_lb_set) & isfinite(obs_ub_set);

if ~any(valid)
    return;
end

t_valid = t_grid(valid);
lb_valid = obs_lb_set(valid);
ub_valid = obs_ub_set(valid);

num_valid = length(t_valid);

if num_valid == 0
    return;
end

if num_valid == 1
    % 只有一个有效 ST 点时，不能使用 interp1。
    if abs(t - t_valid(1)) > single_t_window
        return;
    end

    obs_lb = lb_valid(1);
    obs_ub = ub_valid(1);
else
    if t < t_valid(1) || t > t_valid(end)
        return;
    end

    obs_lb = interp1(t_valid, lb_valid, t, 'linear');
    obs_ub = interp1(t_valid, ub_valid, t, 'linear');
end

if isfinite(obs_lb) && isfinite(obs_ub)
    if obs_ub < obs_lb
        temp = obs_lb;
        obs_lb = obs_ub;
        obs_ub = temp;
    end

    % 防止障碍物边界退化成一个点。
    if obs_ub - obs_lb < obs_min_width
        obs_center = 0.5 * (obs_lb + obs_ub);
        obs_lb = obs_center - 0.5 * obs_min_width;
        obs_ub = obs_center + 0.5 * obs_min_width;
    end

    has_obs = true;
end

end

%% 线性插值，两端采用保持策略
function yq = interpHold(x, y, xq)

yq = zeros(size(xq));

if numel(x) == 1
    yq(:) = y(1);
    return;
end

for i = 1:numel(xq)
    if xq(i) <= x(1)
        yq(i) = y(1);
    elseif xq(i) >= x(end)
        yq(i) = y(end);
    else
        yq(i) = interp1(x, y, xq(i), 'linear');
    end
end

end

%% 根据 DP 曲线估计动力学可达参考点，并在硬边界内修复可行域
function [s_lb, s_ub] = repairReachableCorridor( ...
    s_lb, s_ub, s_dp, hard_lb, hard_ub, ...
    acc_min, acc_max, min_width, s_floor, front_margin)

n = length(s_lb);
dt = 0.5;

s_ref = zeros(n,1);
v_ref = zeros(n,1);

s_ref(1) = s_dp(1);
v_ref(1) = max(0, s_dp(1) / dt);

for i = 2:n
    v_des = (s_dp(i) - s_ref(i-1)) / dt;

    v_low = max(0, v_ref(i-1) + acc_min * dt);
    v_high = max(v_low, v_ref(i-1) + acc_max * dt);

    v_ref(i) = min(max(v_des, v_low), v_high);
    s_ref(i) = s_ref(i-1) + v_ref(i) * dt;
end

for i = 1:n
    [s_lb(i), s_ub(i)] = repairCorridorInsideHardBounds( ...
        s_lb(i), s_ub(i), s_ref(i), hard_lb(i), hard_ub(i), ...
        s_floor, front_margin, min_width);
end

end

%% 根据横向加速度限制计算速度上界
% 当前主函数暂时没有启用该函数，保留用于后续恢复曲率限速。
function s_dot_ub = calcSpeedUpperBound(trajectory_kappa_init, max_lateral_accel, default_speed_ub, n)

s_dot_ub = ones(n,1) * default_speed_ub;

if ~isfinite(max_lateral_accel) || max_lateral_accel <= 0
    return;
end

for i = 1:n
    if i <= length(trajectory_kappa_init)
        kappa = abs(trajectory_kappa_init(i));

        if isfinite(kappa) && kappa > 1e-6
            v_max = sqrt(max_lateral_accel / kappa);

            if isfinite(v_max)
                s_dot_ub(i) = min(default_speed_ub, v_max);
            end
        end
    end

    if s_dot_ub(i) < 1.0
        s_dot_ub(i) = 1.0;
    end
end

end

== matlab function planner_contral/decision_planning/EMplanner/generate st graph_base ==
  data: static_obs_s input; static_obs_l input; static_obs_heading input; dynamic_obs_s_set input; dynamic_obs_l_set input; dynamic_obs_heaidng_set input; static_obs_st_s_lb_set output; tra_s input; tra_l input; tra_path_indexs input; static_obs_st_s_ub_set output; dynamic_obs_st_s_lb_set output; dynamic_obs_st_s_ub_set output; obs_st_t_lb_set output; obs_st_t_ub_set output; static_obs_st_t_lb_set output; static_obs_st_t_ub_set output; plan_s_dot input; plan_l input; plan_s input; dynamic_obs_s_dot input; dynamic_obs_st_t_lb_set output; dynamic_obs_st_t_ub_set output
function [static_obs_st_s_lb_set,static_obs_st_s_ub_set,dynamic_obs_st_s_lb_set,dynamic_obs_st_s_ub_set,obs_st_t_lb_set,obs_st_t_ub_set,static_obs_st_t_lb_set,static_obs_st_t_ub_set,dynamic_obs_st_t_lb_set,dynamic_obs_st_t_ub_set] = ...
    fcn(static_obs_s,static_obs_l,static_obs_heading,dynamic_obs_s_set,dynamic_obs_l_set,dynamic_obs_heaidng_set,tra_s,tra_l,tra_path_indexs,plan_s_dot,plan_l,plan_s,dynamic_obs_s_dot)
% 该函数将生成st图，
%初始化函数变量
coder.extrinsic("plot","axis","figure","drawnow","cla","fill");
% coder.extrinsic('fill');
n = 81;
static_obs_st_s_lb_set=ones(n,1)*inf;
static_obs_st_s_ub_set=ones(n,1)*-inf;
dynamic_obs_st_s_lb_set=ones(n,1)*inf;
dynamic_obs_st_s_ub_set=ones(n,1)*-inf;
% obs_st_t_lb_set=ones(80,1);
% obs_st_t_ub_set=ones(80,1);
t_dynamic=0;
static_obs_st_t_lb_set=(0:0.1:8)';
static_obs_st_t_ub_set=(0:0.1:8)';
dynamic_obs_st_t_lb_set=(0:0.1:8)';
dynamic_obs_st_t_ub_set=(0:0.1:8)';
obs_st_t_lb_set=(0:0.1:8)';
obs_st_t_ub_set=(0:0.1:8)';
%计算静态障碍物的s_lb，s_ub
 [static_obs_lb_,static_obs_ub_,static_obs_t_lb,static_obs_t_ub]=getStaticBound(static_obs_s,static_obs_l,static_obs_heading,tra_s,tra_l,tra_path_indexs,n,plan_s_dot,plan_l,plan_s);
 static_obs_st_s_lb_set=static_obs_lb_;
 static_obs_st_s_ub_set=static_obs_ub_;
%  static_obs_st_t_lb_set=static_obs_t_lb;
%  static_obs_st_t_ub_set=static_obs_t_ub;
[dynamic_obs_lb_,dynamic_obs_ub_,t,dynaimc_obs_t_lb,dynaimc_obs_t_ub]=getDynamicBound(dynamic_obs_s_set,dynamic_obs_l_set,dynamic_obs_heaidng_set,tra_s,tra_l,tra_path_indexs,n,plan_s_dot,plan_l,plan_s,dynamic_obs_s_dot);
dynamic_obs_st_s_lb_set=dynamic_obs_lb_;
dynamic_obs_st_s_ub_set=dynamic_obs_ub_;
% dynamic_obs_st_t_lb_set=dynaimc_obs_t_lb;
% dynamic_obs_st_t_ub_set=dynaimc_obs_t_ub;
t_dynamic=t;



end



function [static_obs_lb,static_obs_ub, static_obs_t_lb,static_obs_t_ub]=getStaticBound(static_obs_s,static_obs_l,static_obs_heading,tra_s,tra_l,index2s,n,plan_s_dot,plan_l,plan_s)
%定义车辆尺寸参数
  vehLength = 5;
  vehWidth = 2;
  vehHalfWidth = vehWidth/2;
%初始化矩阵
  static_obs_lb=ones(n,1)*inf;
  static_obs_ub=ones(n,1)*-inf;
  static_obs_t_lb=(0:0.1:8)';
  static_obs_t_ub=(0:0.1:8)';
  VehPoints = zeros(4,2);       %车辆四个角点坐标
%遍历所有障碍物的s，l
  for i=1:length(static_obs_s)
     if isnan(static_obs_s(i))
         break
     end
     if abs(plan_l-static_obs_l(i))>2
         continue
     end
     %如果不为空，执行下一步动作
     for j=1:n
     %获取车辆信息
     %先计算t
     t=(static_obs_s(i)-plan_s)/plan_s_dot;
     if j<t/0.1
         continue
     end
     static_obs_t_lb(j)=t;    %静态障碍物出现的时间
     static_obs_t_ub(j)=t;
     rear_s=static_obs_s(i);  %静态障碍物此刻的L
     rear_l=static_obs_l(i);
     heading=static_obs_heading(i);
     %转换前轴坐标信息
     front_s=rear_s+vehLength*cos(heading);
     front_l=rear_l+vehLength*sin(heading);
     % 根据前后中心点、航向角计算目障碍车四个轮廓点位置（顺时针编号）
     VehPoints(1,1) = rear_s - vehHalfWidth * sin(heading);
     VehPoints(1,2) = rear_l + vehHalfWidth * cos(heading);
     VehPoints(2,1) = front_s - vehHalfWidth * sin(heading);
     VehPoints(2,2) = front_l + vehHalfWidth * cos(heading);
     VehPoints(3,1) = front_s + vehHalfWidth * sin(heading);
     VehPoints(3,2) = front_l - vehHalfWidth * cos(heading);
     VehPoints(4,1) = rear_s + vehHalfWidth * sin(heading);
     VehPoints(4,2) = rear_l - vehHalfWidth * cos(heading);
     %计算四个角点相对与轨迹最近的索引值
     index_matrix=zeros(4,1);
     dist_matrix=zeros(4,1);
     for z=1:4
        dist=inf;
        index=0;
        for k=1:length(tra_s)
            if isnan(tra_s(k))
                break
            end
        %开始计算四个角点距离轨迹的最大最小索引值
          dist_s=tra_s(k)-VehPoints(z,1);
          dist_l=tra_l(k)-VehPoints(z,2);
          dist_temp=sqrt(dist_s^2+dist_l^2);
          if dist_temp<dist
              dist=dist_temp;
              index=k;
          end
        end
        index_matrix(z,1)=index;
        dist_matrix(z,1)=dist;
     end
     index_sort=sort(index_matrix,"descend");
     min_index=index_sort(4,1);
     max_index=index_sort(1,1);
     static_obs_lb(j) =index2s( min_index);
     static_obs_ub(j) = index2s(max_index);
     end
  end
 
 end


%计算动态障碍物的s_lb,s_ub  ,plan_s_dot,plan_l,plan_s,dynamic_obs_s_dot);
function [dynamic_obs_lb,dynamic_obs_ub,t,dynaimc_obs_t_lb,dynaimc_obs_t_ub]=getDynamicBound(dynamic_obs_s,dynamic_obs_l,dynamic_obs_heading,tra_s,tra_l,index2s,n,plan_s_dot,plan_l,plan_s,obs_s_dot)
%定义车辆尺寸参数
  vehLength = 5;
  vehWidth = 2;
  vehHalfWidth = vehWidth/2;
%初始化矩阵
   t=0;
  dynamic_obs_lb=ones(n,1)*inf;
  dynamic_obs_ub=ones(n,1)*-inf;
  dynaimc_obs_t_lb=(0:0.1:8)';
  dynaimc_obs_t_ub=(0:0.1:8)';
  VehPoints = zeros(4,2);  %车辆四个角点坐标
  for i=1:length(dynamic_obs_s)
     if isnan(dynamic_obs_s(i))
         break;
     end
     if abs(plan_l-dynamic_obs_l(i))>2
         continue
     end
     %计算障碍物的相对时间
  
     for  j=1:n
       t=(dynamic_obs_s(i)-plan_s)/(plan_s_dot);
      if j<t/0.1
         continue
      else
       dynaimc_obs_t_lb(j)=t;
       dynaimc_obs_t_ub(j)=t;
       break
      end
     end

     rear_s=dynamic_obs_s(i);
     rear_l=dynamic_obs_l(i);
   
     heading=dynamic_obs_heading(i);
     %转换前轴坐标信息
     front_s=rear_s+vehLength*cos(heading);
     front_l=rear_l+vehLength*sin(heading);
     % 根据前后中心点、航向角计算目障碍车四个轮廓点位置（顺时针编号）
     VehPoints(1,1) = rear_s - vehHalfWidth * sin(heading);
     VehPoints(1,2) = rear_l + vehHalfWidth * cos(heading);
     VehPoints(2,1) = front_s - vehHalfWidth * sin(heading);
     VehPoints(2,2) = front_l + vehHalfWidth * cos(heading);
     VehPoints(3,1) = front_s + vehHalfWidth * sin(heading);
     VehPoints(3,2) = front_l - vehHalfWidth * cos(heading);
     VehPoints(4,1) = rear_s + vehHalfWidth * sin(heading);
     VehPoints(4,2) = rear_l - vehHalfWidth * cos(heading);
     %计算四个角点相对与轨迹最近的索引值
     index_matrix=zeros(4,1);
     dist_matrix=zeros(4,1);
     for z=1:4
        dist=inf;
        index=0;
        for k=1:length(tra_s)
            if isnan(tra_s(k))
                break
            end
        %开始计算四个角点距离轨迹的最大最小索引值
          dist_s=tra_s(k)-VehPoints(z,1);
          dist_l=tra_l(k)-VehPoints(z,2);
          dist_temp=sqrt(dist_s^2+dist_l^2);
          if dist_temp<dist
              dist=dist_temp;
              index=k;
          end
        end
        index_matrix(z,1)=index;
        dist_matrix(z,1)=dist;
     end
     index_sort=sort(index_matrix,"descend");
     min_index=index_sort(4,1);
     max_index=index_sort(1,1);
     dynamic_obs_lb(j) =index2s( min_index);
     dynamic_obs_ub(j) = index2s(max_index);
   end
end
